simulink model "PVarray"  (R2023b)
settings: Solver=VariableStepAuto  StartTime=0.0  StopTime=15  RelTol=1e-3
libraries: powerlib x4, re_lib x1
settings Model: Creator=26454  LastModifiedBy=26454
settings SolverCC: AlgebraicLoopSolver=LineSearch
settings DebuggingCC: UnconnectedInputMsg=warning  UnconnectedOutputMsg=warning  UnconnectedLineMsg=warning
settings ModelReferenceCC: EnableRefExpFcnMdlSchedulingChecks=on

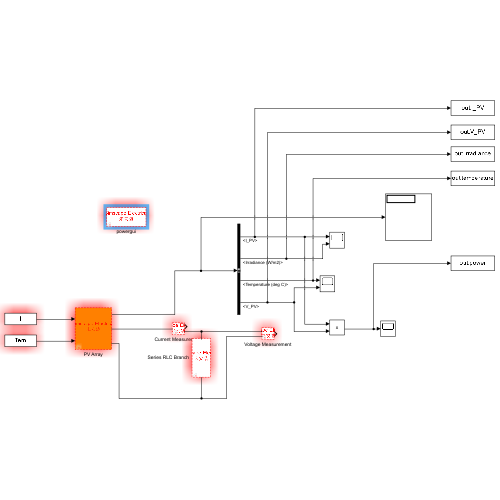
[thumbnail: Simulink's stored preview of the top-level diagram]
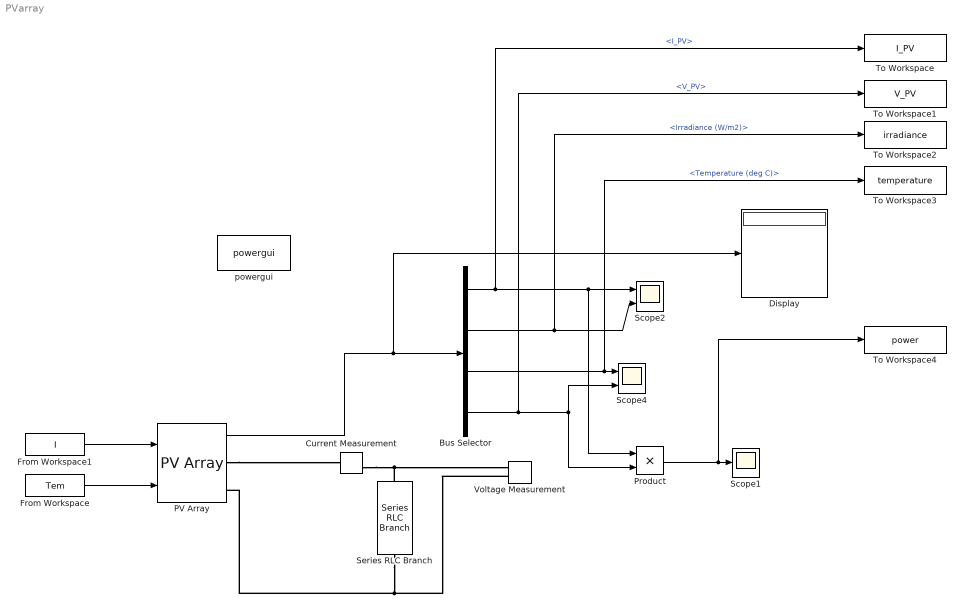
== system PVarray ==
  Bus Selector : BusSelector  OutputSignals=I_PV,Irradiance (W/m2),Temperature (deg C),V_PV
  Current Measurement : powerlib/Measurements/Current Measurement  PhasorSimulation=off  OutputType=Complex  PSBequivalent=0
  Display : Display
  From Workspace : FromWorkspace  VariableName=Tem  OutDataTypeStr=double  SampleTime=1e-5
  From Workspace1 : FromWorkspace  VariableName=I  OutDataTypeStr=double  SampleTime=1e-5
  PV Array : re_lib/Solar/PV Array  Npar=100  Nser=100  PlotType=array @ 1000 W/m2 & specified temperatures  S_vec="[ 1000  500  100 ]"  Temp_C_vec="[ 45 25  ]"  ModuleName=Schuco USA MPE 360 AL 01  PlotWhenSelected=off  Pm=359.331  Ncell=216  Voc=191.1  Isc=3.02  Vm=149.1  Im=2.41  beta_Voc_pc=-0.349  alpha_Isc_pc=0.096987  beta_Voc=-0.66694  alpha_Isc=0.002929  IL=3.0973  I0=7.0809e-11  nI=1.4191  Rsh=293.7864  Rs=7.523  RobustModel=off  RobustCellTemperature=25  BAL=off  Tc=1e-6  Tfilter=5e-5
  Product : Product
  Scope1 : Scope
  Scope2 : Scope  NumInputPorts=2
  Scope4 : Scope  NumInputPorts=2
  Series RLC Branch : powerlib/Elements/Series RLC Branch  LConnTagsString=__new0  RConnTagsString=__new0  BranchType=R  Resistance=10  Inductance=1e-3  SetiL0=off  InitialCurrent=0  Capacitance=1e-6  Setx0=off  InitialVoltage=0  Measurements=None
  To Workspace : ToWorkspace  VariableName=I_PV  SampleTime=-1
      settings: Decimation=100  Save2DSignal=2-D array (concatenate along first dimension)
  To Workspace1 : ToWorkspace  VariableName=V_PV  SampleTime=-1
      settings: Decimation=100  Save2DSignal=2-D array (concatenate along first dimension)
  To Workspace2 : ToWorkspace  VariableName=irradiance  SampleTime=-1
      settings: Decimation=100  Save2DSignal=2-D array (concatenate along first dimension)
  To Workspace3 : ToWorkspace  VariableName=temperature  SampleTime=-1
      settings: Decimation=100  Save2DSignal=2-D array (concatenate along first dimension)
  To Workspace4 : ToWorkspace  VariableName=power  SampleTime=-1
      settings: Decimation=100  Save2DSignal=2-D array (concatenate along first dimension)
  Voltage Measurement : powerlib/Measurements/Voltage Measurement  PhasorSimulation=off  OutputType=Complex  PSBequivalent=0
  powergui : powerlib/powergui  Priority=1  SimulationMode=Discrete  SampleTime=1e-5  frequency=60  Iterations=50  frequencyindice=0  Pbase=100e6  ErrMax=1e-4  UnitsV=kV  UnitsW=MW  buscounter=0  FunctionMessages=off  echomessages=off  EnableUseOfTLC=off  CurrentSourceSwitches=off  DisableSnubberDevices=off  DisableRonSwitches=off  DisableVfSwitches=off  DisplayEquations=off  AutomaticDiscreteSolvers=off  SolverType=Tustin/Backward Euler (TBE)  Interpol=off  ExternalGateDelay=off  methode=off  Ts=100  x0status=blocks  SPID=on  SwTol=0  HookPort=off  NonlinearTolerance=1e-4  nMaxIteration=100  ContinueOnMaxIteration=off  RestoreLinks=warning  ResistiveCurrentMeasurement=off  Frange=[0:2:500]  Ylog=off  Xlog=on  ShowGrid=off  save=off  variable=ZData  structure=0  ZoomFFT=off  StartTime=0.0  cycles=1  DisplayStyle=1  fundamental=60  FreqAxis=off  MaxFrequency=1000  frequencyindicesteady=1  RmsSteady=1  display=off
  wires:
  PV Array/1 -> Display/1, Bus Selector/1
  From Workspace1/1 -> PV Array/1
  From Workspace/1 -> PV Array/2
  Bus Selector/1 -> Scope2/1, Product/1, To Workspace/1  "<I_PV>"
  Bus Selector/2 -> To Workspace2/1, Scope2/2  "<Irradiance (W/m2)>"
  Bus Selector/3 -> To Workspace3/1, Scope4/1  "<Temperature (deg C)>"
  Bus Selector/4 -> To Workspace1/1, Scope4/2, Product/2  "<V_PV>"
  Product/1 -> To Workspace4/1, Scope1/1
  connections:
  PV Array/RConn1 -- Current Measurement/LConn1
  Current Measurement/RConn1 -- Series RLC Branch/LConn1 -- Voltage Measurement/LConn1
  Voltage Measurement/LConn2 -- Series RLC Branch/RConn1 -- PV Array/RConn2
